simulink model "Child_App"  (R2023a)
settings: Solver=FixedStepDiscrete  StartTime=0.0  StopTime=inf  RelTol=1e-3
libraries: androiduilib x11, androidcommunicationlib x6, androidsensorlib x4, androidaudiovideolib x4
settings Model: Creator=parag  LastModifiedBy=parag
settings OptimizationCC: EnhancedBackFolding=on  PassReuseOutputArgsAs=Individual arguments  ZeroExternalMemoryAtStartup=off  ZeroInternalMemoryAtStartup=off  MaxStackSize=64  OptimizeBlockOrder=speed  DifferentSizesBufferReuse=on  OptimizationCustomize=off  EfficientTunableParamExpr=on
settings DebuggingCC: ParameterTunabilityLossMsg=error
settings HardwareCC: ProdBitPerPointer=32  ProdBitPerSizeT=32  ProdBitPerPtrDiffT=32  ProdLargestAtomicInteger=Long  ProdLargestAtomicFloat=Double  ProdWordSize=32  ProdHWDeviceType=ARM Compatible->ARM Cortex  UseEmbeddedCoderFeatures=off  UseSimulinkCoderFeatures=off
settings SFSimCC: MATLABDynamicMemAlloc=off
settings RTWCC: Description=Embedded Coder  SystemTargetFile=ert.tlc  HardwareBoard=Android Device  TLCOptions="-aInlineSetEventsForThisBaseRateFcn=TLC_FALSE -aSuppressMultiTaskScheduler=TLC_FALSE  -aRateBasedStepFcn=0"  TemplateMakefile=ert_default_tmf  RTWVerbose=off  Toolchain=Android SDK/NDK Tools
settings CodeAppCC: ForceParamTrailComments=on  IgnoreCustomStorageClasses=off  OperatorAnnotations=on  SimulinkDataObjDesc=on  SFDataObjDesc=on  InsertBlockDesc=on
settings ERTTargetCC: SupportNonInlinedSFcns=on

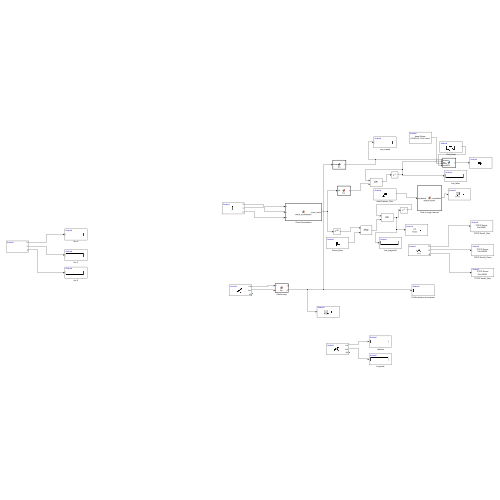
[thumbnail: Simulink's stored preview of the top-level diagram]
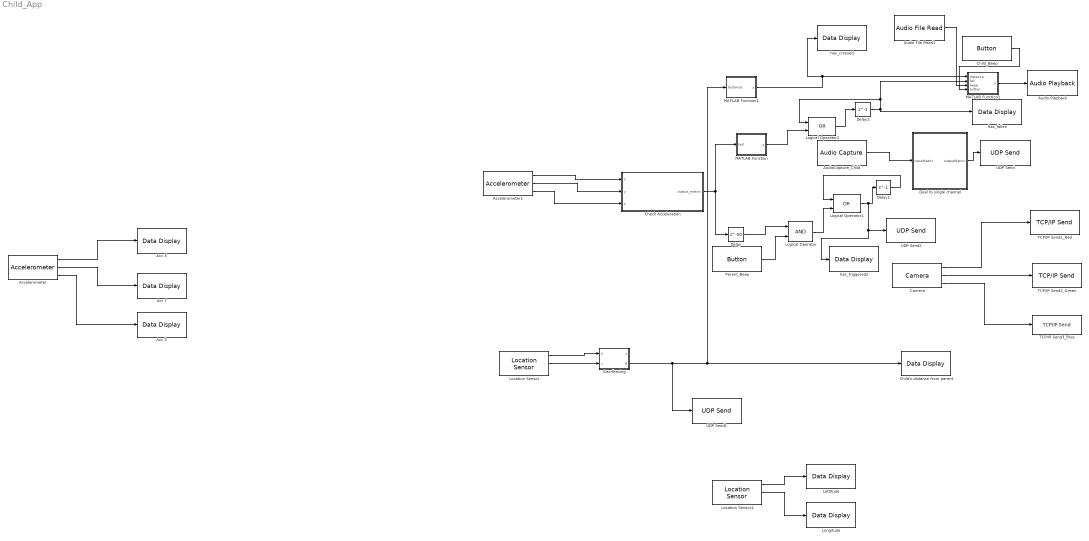
== system Child_App ==
  Acc X : androiduilib/Data Display  DataDisplayId=Child_App/Acc_X  Format=Float  Precision=6  SimulateUsing=Code generation  blockPlatform=Android
  Acc Y : androiduilib/Data Display  DataDisplayId=Child_App/Acc_Y  Format=Float  Precision=6  SimulateUsing=Code generation  blockPlatform=Android
  Acc Z : androiduilib/Data Display  DataDisplayId=Child_App/Acc_Z  Format=Float  Precision=6  SimulateUsing=Code generation  blockPlatform=Android
  Accelerometer : androidsensorlib/Accelerometer  OutputVector=off  SampleTime=0.1  BlockPlatform=Android
  Accelerometer1 : androidsensorlib/Accelerometer  OutputVector=off  SampleTime=0.1  BlockPlatform=Android
  Audio File Read1 : androidaudiovideolib/Audio File Read  FileName=C:\Users\parag\Downloads\beep-04.wav  FrameSize=4410
  Audio Playback : androidaudiovideolib/Audio Playback  SampleFreq=44100  AudioSamplingFreq=44100  SampleTime=0.1  DeviceStr=0  QueueDuration=0  BlockPlatform=Android
  AudioCapture_Child : androidaudiovideolib/Audio Capture  SampleFreq=44100  FrameSize=4410  SampleTime=0.1  SimulateUsing=Code generation  DeviceStr=0  QueueDuration=0  BlockPlatform=Android  AudioSamplingFreq=44100
  Camera : androidaudiovideolib/Camera  CameraLocation=Back  CameraResolutions=Back - 640x480  Width=640  Height=480  SampleTime=2  BlockPlatform=Android
  Check Acceleration : MATLAB Function  TreatAsAtomicUnit=on
  Child's distance from parent : androiduilib/Data Display  DataDisplayId=Child_App/Child's_distance_from_parent  Format=Float  Precision=6  SimulateUsing=Code generation  blockPlatform=Android
  Child_Beep : androiduilib/Button  ButtonState=Pressed  ButtonId=Child_App/Child_Beep  State=on  SampleTime=0.1  BlockPlatform=Android
  Delay : Delay  DelayLength=50  InitialCondition=0
  Delay1 : Delay  DelayLength=1
  Delay2 : Delay  DelayLength=1
  Dual to single channel : MATLAB Function  TreatAsAtomicUnit=on
  Geo-fencing : MATLAB Function  TreatAsAtomicUnit=on
  Lattitude : androiduilib/Data Display  DataDisplayId=Child_App/Lattitude  Format=Float  Precision=6  SimulateUsing=Code generation  blockPlatform=Android
  Location Sensor : androidsensorlib/Location Sensor  OutputVector=off  SampleTime=0.1  BlockPlatform=Android
  Location Sensor1 : androidsensorlib/Location Sensor  OutputVector=off  SampleTime=0.1  BlockPlatform=Android
  Logical Operator : Logic  AllPortsSameDT=off  OutDataTypeStr=boolean
  Logical Operator1 : Logic  Operator=OR  AllPortsSameDT=off  OutDataTypeStr=boolean
  Logical Operator2 : Logic  Operator=OR  AllPortsSameDT=off  OutDataTypeStr=boolean
  Longitude : androiduilib/Data Display  DataDisplayId=Child_App/Longitude  Format=Float  Precision=6  SimulateUsing=Code generation  blockPlatform=Android
  MATLAB Function : MATLAB Function  TreatAsAtomicUnit=on
  MATLAB Function1 : MATLAB Function  TreatAsAtomicUnit=on
  MATLAB Function2 : MATLAB Function  TreatAsAtomicUnit=on
  Parent_Beep : androiduilib/Button  ButtonState=Pressed  ButtonId=Child_App/Parent_Beep  State=on  SampleTime=0.1  BlockPlatform=Android
  TCP/IP Send1_Red : androidcommunicationlib/TCP//IP Send  TCPSendId=Child_App/TCP//IP_Send1_Red  Mode_=Server  LocalServerPort_=25001  RemoteAddr_=127.0.0.1  RemoteServerPort_=25000  ClientPortBindingSelection_=off  ClientPortToBind_=35000  BlockingMode_=off  BlockTimeout_=0.1
  TCP/IP Send2_Green : androidcommunicationlib/TCP//IP Send  TCPSendId=Child_App/TCP//IP_Send2_Green  Mode_=Server  LocalServerPort_=25002  RemoteAddr_=127.0.0.1  RemoteServerPort_=25002  ClientPortBindingSelection_=off  ClientPortToBind_=35000  BlockingMode_=off  BlockTimeout_=0.1
  TCP/IP Send3_Blue : androidcommunicationlib/TCP//IP Send  TCPSendId=Child_App/TCP//IP_Send3_Blue  Mode_=Server  LocalServerPort_=25003  RemoteAddr_=127.0.0.1  RemoteServerPort_=25000  ClientPortBindingSelection_=off  ClientPortToBind_=35000  BlockingMode_=off  BlockTimeout_=0.1
  UDP Send : androidcommunicationlib/UDP Send  remoteURL='10.7.5.27'  remotePort=25011  localURL='0.0.0.0'  localPortSource=Automatically determine  localPort=-1  sampletime=-1  blockPlatform=Android  separateLengthPort=0
  UDP Send1 : androidcommunicationlib/UDP Send  remoteURL='10.7.5.27'  remotePort=25009  localURL='0.0.0.0'  localPortSource=Automatically determine  localPort=-1  sampletime=-1  blockPlatform=Android  separateLengthPort=0
  UDP Send2 : androidcommunicationlib/UDP Send  remoteURL='10.7.5.27'  remotePort=25010  localURL='0.0.0.0'  localPortSource=Automatically determine  localPort=-1  sampletime=-1  blockPlatform=Android  separateLengthPort=0
  has_crossed : androiduilib/Data Display  DataDisplayId=Child_App/has_crossed  Format=Float  Precision=6  SimulateUsing=Code generation  blockPlatform=Android
  has_fallen : androiduilib/Data Display  DataDisplayId=Child_App/has_fallen  Format=Float  Precision=6  SimulateUsing=Code generation  blockPlatform=Android
  has_triggered2 : androiduilib/Data Display  DataDisplayId=Child_App/has_triggered2  Format=Float  Precision=6  SimulateUsing=Code generation  blockPlatform=Android
  wires:
  Parent_Beep/1 -> Logical Operator/2
  Delay1/1 -> Logical Operator1/1
  Camera/1 -> TCP/IP Send1_Red/1
  Camera/2 -> TCP/IP Send2_Green/1
  Camera/3 -> TCP/IP Send3_Blue/1
  MATLAB Function1/1(y) -> MATLAB Function2/1(distance), has_crossed/1
  Dual to single channel/1(outputMatrix) -> UDP Send/1
  MATLAB Function2/1(y) -> Audio Playback/1
  Accelerometer/1 -> Acc X/1
  Delay2/1 -> MATLAB Function2/2(fall), Logical Operator2/1, has_fallen/1
  Audio File Read1/1 -> MATLAB Function2/3(beep)
  Accelerometer/2 -> Acc Y/1
  Logical Operator1/1 -> Delay1/1, has_triggered2/1, UDP Send2/1
  MATLAB Function/1(y) -> Logical Operator2/2
  Logical Operator2/1 -> Delay2/1
  Logical Operator/1 -> Logical Operator1/2
  Accelerometer/3 -> Acc Z/1
  Location Sensor/2 -> Geo-fencing/2(v)
  Location Sensor/1 -> Geo-fencing/1(u)
  Geo-fencing/2(d) -> UDP Send1/1, Child's distance from parent/1, MATLAB Function1/1(distance)
  Location Sensor1/2 -> Longitude/1
  AudioCapture_Child/1 -> Dual to single channel/1(inputMatrix)
  Check Acceleration/1(output_matrix) -> Delay/1, MATLAB Function/1(fall)
  Accelerometer1/2 -> Check Acceleration/2(y)
  Accelerometer1/3 -> Check Acceleration/3(z)
  Delay/1 -> Logical Operator/1
  Accelerometer1/1 -> Check Acceleration/1(x)
  Location Sensor1/1 -> Lattitude/1
  Child_Beep/1 -> MATLAB Function2/4(button)

== matlab function Child_App/MATLAB Function1 ==
  data: distance input; y output
function y = fcn(distance)
    if distance > 0.08 ;
            y = 1;
    else ;
        y = 0;
    end ;
end

== matlab function Child_App/Geo-fencing ==
  data: u input; y output; v input; d output
function [y,d] = fcn(u, v)
N = 4410;
freq = 600;

% Calculate the sampling frequency needed for a 10-second duration
duration = 10;  % Duration in seconds
Fs = N / duration;

% Generate a time vector
t = (0:N-1) / Fs;

% Generate the sine wave
sound_array = zeros(N, 2, 'int16');
khali = zeros(N, 2, 'int16');
%starts N x 2 matrix
sound_array(:,1) = int16(sin(2*pi*freq*t));
sound_array(:,2) = int16(sin(2*pi*freq*t));

% Define the center of the circle
center_lat = 23.210336;  % Latitude of the center
center_lon = 72.683842;  % Longitude of the center

% Define the radius of the circle (you need to set this value)
radius_km = 0.08;  % Replace with the desired radius in kilometers

% Earth's mean radius in kilometers
earth_radius_km = 6371;

% Convert latitude and longitude from degrees to radians
center_lat_rad = deg2rad(center_lat);
center_lon_rad = deg2rad(center_lon);
point_lat_rad = deg2rad(u);
point_lon_rad = deg2rad(v);

% Calculate the Haversine distance between the center and the point
dlat = point_lat_rad - center_lat_rad;
dlon = point_lon_rad - center_lon_rad;

a = sin(dlat/2)^2 + cos(center_lat_rad) * cos(point_lat_rad) * sin(dlon/2)^2;
c = 2 * atan2(sqrt(a), sqrt(1 - a));
distance_km = earth_radius_km * c;
d = distance_km  ;
% Check if the point is inside the circle
if distance_km >= radius_km
    y = 1;
else
    y = 0;
end
end

== matlab function Child_App/MATLAB Function ==
  data: y output; fall input
function y = fcn(fall)
    if fall == 1 ; 
        y = 1;
    else ;
        y = 0;
    end ;
end

== matlab function Child_App/Dual to single channel ==
  data: inputMatrix input; outputMatrix output
function outputMatrix = selectColumn(inputMatrix)
    outputMatrix = inputMatrix(:,1);
end

== matlab function Child_App/MATLAB Function2 ==
  data: distance input; y output; fall input; beep input; button input
function y = fcn(distance,fall,beep,button)
    if distance || fall == 1 ; 
        y = [beep,beep];
    else ;
        y = zeros(4410,2,'int16');
    end ;
    if button == 0 ;
        y = zeros(4410,2,'int16');
end

== matlab function Child_App/Check Acceleration ==
  data: x input; output_matrix output; y input; z input
function output_matrix  = check_acceleration(x, y, z)
    resultant_acceleration = sqrt(x^2 + y^2 + z^2);
    output_matrix = resultant_acceleration > 15;
end
